simulink model "exo1"  (R2015b)
settings: Solver=VariableStepAuto  StartTime=0.0  StopTime=10.0  RelTol=1e-3
values from neighbouring files (symbols this model uses):
  H = H*Ki/s    [ex3.m]    (also in ex4.m = K*exp(-Tr*s)/(0.5*s+1))
  Tr = 0.5    [ex4.m]
settings Model: Creator=max.sonzogni  LastModifiedBy=max.sonzogni

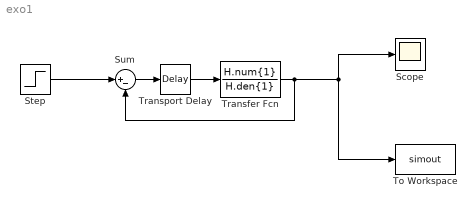
== system exo1 ==
  Scope : Scope
  Step : Step  SampleTime=0
  Sum : Sum  Inputs=|+-
  To Workspace : ToWorkspace  VariableName=simout  SaveFormat=Structure With Time  SampleTime=-1
  Transfer Fcn : TransferFcn  Numerator=H.num{1}  Denominator=H.den{1}
  Transport Delay : TransportDelay  DelayTime=Tr
  wires:
  Step/1 -> Sum/1
  Transfer Fcn/1 -> Scope/1, To Workspace/1, Sum/2
  Sum/1 -> Transport Delay/1
  Transport Delay/1 -> Transfer Fcn/1
